simulink library "PCMULib"  (R2022b)
settings: Solver=ode45  StartTime=0.0  StopTime=10.0  RelTol=1e-3  EnableMultiTasking=on
undefined symbols (not defined in the file or in its folder): BreakpointData, BreakpointData1, BreakpointData2, BreakpointData_One_A, BreakpointData_Two_A, caaaa_dbi, caaaa_swi, cTmComprCtrl_n_i16SM4CmpHeatKiMax, cTmComprCtrl_n_i16SM4CmpHeatKiMin, cTmComprCtrl_n_i16SM4CmpHeatKpMax, cTmComprCtrl_n_i16SM4CmpHeatKpMin, cTmComprCtrl_Te_s32ErrCmpPIContinueHeatH, cTmComprCtrl_Te_s32ErrCmpPIContinueHeatL, cTmIn_n_ElacCmprReq_db, cTmIn_n_ElacCmprReq_sw, db, dbi, E2E_P01DataIDMode, E2E_P01ReceiverStatusType, EnumClass, iBit, initalValue, No_Runnable_Period, ObB_EidBsgStDerat_C, p_OVERRIDE_MASTER_SWITCH, SlDemoSign, sw, swi, SwitchOff_P, SwitchOn_P, Table, TableData_M, VCCTi33, VSysD_FidVehDerat1_C
libraries: simulink x22, CCMLib x11, simulink_need_slupdate x9, UXFD_Lib x7, canmsglib x2, PTCC_Lib x1, hdlsllib x1
(part 4 of 7)

== system PCMULib/Standard/Calibration ==
  note: Look-up masks including
      | lookup and prelookup blocks
  note: Look-up and pre-lookup blocks
  note: Calibration
  note: OverRide
  1-D Lookup Table : Lookup  InputValues=BreakpointData  Table=Table  LookUpMeth=Interpolation-Use End Values  OutDataTypeStr=single  SaturateOnIntegerOverflow=off
      settings: CopyFcn=set_param(gcbh,'ShowName','on');
  1-D Lookup Table Without Const_Param : Subsystem  Tag=AVLib calibration  mask(Lookup Table 1D){BlockConfiguration=freeze, BreakpointData=BreakpointData, ReferenceBreakpointData=off, OpenMPTBreakpointData=off, OpenADDBreakpointData=off, IndexSearchMethod=Linear search, Table=Table, ReferenceTable=off, OpenMPTTable=off, OpenADDTable=off, InterpMethod=Linear, DisplayCalibrationNames=off, AdoptBlockName=off, OutMin=[], OutMax=[], OutDataType=Inherit: Inherit from data, IndexDataType=uint8, FractionDataType=Inherit: Inherit via internal rule}
      mask prompts: BlockConfiguration "Block configuration:"; BreakpointData "Breakpoint data:"; ReferenceBreakpointData "Treat as calibration reference"; OpenMPTBreakpointData "Open breakpoint data"; OpenADDBreakpointData "Open ADD breakpoint data"; IndexSearchMethod "Index search method:"; Table "Table data:"; ReferenceTable "Treat as calibration reference"; OpenMPTTable "Open table data"; OpenADDTable "Open ADD table data"; InterpMethod "Interpolation method:"; DisplayCalibrationNames "Block annotation with calibration data"; AdoptBlockName "Adopt block name from table name"; OutMin "Output minimum:"; OutMax "Output maximum:"; OutDataType "Output data type:"; IndexDataType "Index data type:"; FractionDataType "Fraction data type:"
      mask help: Perform 1-D linear interpolation of input values using the specified table.
      mask init:
      | % get and transmit data type from value
      | if strcmp(OutDataType,'Inherit: Inherit from data')
      |   val = Table;  nam = get_param(gcb,'Table');
      |   if evalin('base',['exist(''',nam,''',''var'')']),  s = evalin('base',nam);
      |     if isa(s,'mpt.Parameter') || isa(s,'Simulink.Parameter') || isa(s,'AVLmpt.Parameter')
      |       valDataType = s.DataType;
      |       if strcmp(valDataType,'auto'), valDataType = 'double'; end
      |     else
      |       valDataType = class(s);
      |     end
      |   else
      |       valDataType = class(val);
      |   end
      |   if strcmp(valDataType,'logical'), valDataType = 'boolean'; end
      |   set_param([gcb,'/Curve'],'OutDataTypeStr',valDataType)
      | end
      | if 1
      |   val = BreakpointData;  nam = get_param(gcb,'BreakpointData');
      |   if evalin('base',['exist(''',nam,''',''var'')']),  s = evalin('base',nam);
      |     if isa(s,'mpt.Parameter') || isa(s,'Simulink.Parameter') || isa(s,'AVLmpt.Parameter')
      |       valDataType = s.DataType;
      |       if strcmp(valDataType,'auto'), valDataType = 'double'; end
      |     else
      |       valDataType = class(s);
      |     end
      |   else
      |       valDataType = class(val);
      |   end
      |   if strcmp(valDataType,'logical'), valDataType = 'boolean'; end
      |   set_param([gcb,'/u'],'OutDataTypeStr',valDataType)
      | end
      | 
      | % © AVL S&F, C.A. Roduner, Nov/18/2009
      | if BlockConfiguration==1 && (~strcmp(get_param(gcb,'LinkStatus'),'resolved') ...
      |   || (~strncmp(get_param(gcb,'Referenceblock'),'AVLib',5) && ~exist('AVLib_Init','file') ) ), return, end
      | AVLib_Init( 'LookupTable1D_init', gcb, ...
      |   BlockConfiguration,IndexSearchMethod,InterpMethod, ...
      |   DisplayCalibrationNames,AdoptBlockName,  ...
      |   BreakpointData,ReferenceBreakpointData,OpenMPTBreakpointData, OpenADDBreakpointData, ...
      |   Table,ReferenceTable,OpenMPTTable,OpenADDTable, ...
      |   IndexDataType, FractionDataType, ...
      |   OutMin,OutMax,OutDataType ...
      | );
      mask Help: eval('try openDocu(gcb), catch try run([fileparts(which(''AVLib'')),''\..\AVLibDocu\openDocu'']), catch errordlg(''No documentation available on Matlab path.'',gcb,''modal''), end, end')
      mask TypeOptions BlockConfiguration: freeze | enable | default
      mask Callback BreakpointData:
      | if strcmp(get_param(gcb,'BlockConfiguration'),'freeze'), return, end
      | AVLib_Init('Calibration_cb',gcb,'BreakpointData')
      mask Callback OpenMPTBreakpointData:
      | if strcmp(get_param(gcb,'BlockConfiguration'),'freeze'), return, end
      | AVLib_Init('OpenMPT_cb',gcb,'BreakpointData')
      mask Callback OpenADDBreakpointData:
      | if strcmp(get_param(gcb,'BlockConfiguration'),'freeze'), return, end
      | if strcmp(get_param(gcb,'OpenADDBreakpointData'),'on')
      |   set_param(gcb,'OpenADDBreakpointData','off')
      |   set_param(gcb,'BreakpointData', connectADD(get_param(gcb,'BreakpointData'),'axis') )
      | end
      mask TypeOptions IndexSearchMethod: Evenly spaced points | Linear search | Binary search
      mask Callback Table:
      | if strcmp(get_param(gcb,'BlockConfiguration'),'freeze'), return, end
      | AVLib_Init('Calibration_cb',gcb,'Table')
      mask Callback OpenMPTTable:
      | if strcmp(get_param(gcb,'BlockConfiguration'),'freeze'), return, end
      | AVLib_Init('OpenMPT_cb',gcb,'Table')
      mask Callback OpenADDTable:
      | if strcmp(get_param(gcb,'BlockConfiguration'),'freeze'), return, end
      | if strcmp(get_param(gcb,'OpenADDTable'),'on')
      |   set_param(gcb,'OpenADDTable','off')
      |   set_param(gcb,'Table', connectADD(get_param(gcb,'Table'),'curve') )
      | end
      mask TypeOptions InterpMethod: None - Flat | Linear
      mask Callback AdoptBlockName:
      | if strcmp(get_param(gcb,'BlockConfiguration'),'freeze'), return, end
      | AVLib_Init('AdoptBlockName_cb',gcb,get_param(gcb,'Table'))
      mask TypeOptions OutDataType: Inherit: Inherit from data | Inherit: Inherit via back propagation | double | single | int8 | uint8 | int16 | uint16 | int32 | uint32 | boolean
      mask TypeOptions IndexDataType: uint8 | uint16 | uint32
      mask TypeOptions FractionDataType: Inherit: Inherit via internal rule | double | single
      mask DialogControl ParameterTabVar0 Prompt: Main
      mask DialogControl ParameterTabVar01 Prompt: Signal Attributes
      mask DialogControl ParameterTabVar012 Prompt: Lookup Attributes
      mask Display:
      | plot( getfield(get_param(gcb,'UserData'),'xy') )
      | plot( getfield(get_param(gcb,'UserData'),'xy_InterpMethod') )
      | color('blue'), plot( getfield(get_param(gcb,'UserData'),'xy_C') )
  2-D Lookup Table : Lookup2D  RowIndex=BreakpointData1  ColumnIndex=BreakpointData2  Table=Table  LookUpMeth=Interpolation-Use End Values  OutDataTypeStr=single  SaturateOnIntegerOverflow=off  InputSameDT=off
      settings: CopyFcn=set_param(gcbh,'ShowName','on');
  2-D Lookup Table Without Const_Param : Subsystem  Tag=AVLib calibration  mask(Lookup Table 2D){BlockConfiguration=freeze, BreakpointData1=BreakpointData1, ReferenceBreakpointData1=off, OpenMPTBreakpointData1=off, OpenADDBreakpointData1=off, BreakpointData2=BreakpointData2, ReferenceBreakpointData2=off, OpenMPTBreakpointData2=off, OpenADDBreakpointData2=off, IndexSearchMethod=Binary search, Table=Table, ReferenceTable=off, OpenMPTTable=off, OpenADDTable=off, InterpMethod=Linear, DisplayCalibrationNames=off, AdoptBlockName=off, OutMin=[], OutMax=[], OutDataType=Inherit: Inherit from data, IndexDataType=uint8, FractionDataType=Inherit: Inherit via internal rule}
      mask prompts: BlockConfiguration "Block configuration:"; BreakpointData1 "Breakpoint data for 1st input (x-axis, row index):"; ReferenceBreakpointData1 "Treat as calibration reference"; OpenMPTBreakpointData1 "Open breakpoint data 1"; OpenADDBreakpointData1 "Open ADD breakpoint data 1"; BreakpointData2 "Breakpoint data for 2nd input (y-axis, column index):"; ReferenceBreakpointData2 "Treat as calibration reference"; OpenMPTBreakpointData2 "Open breakpoint data 2"; OpenADDBreakpointData2 "Open ADD breakpoint data 2"; IndexSearchMethod "Index search method:"; Table "Table data:"; ReferenceTable "Treat as calibration reference"; OpenMPTTable "Open table data"; OpenADDTable "Open ADD table data"; InterpMethod "Interpolation method:"; DisplayCalibrationNames "Block annotation with calibration data"; AdoptBlockName "Adopt block name from table name"; OutMin "Output minimum:"; OutMax "Output maximum:"; OutDataType "Output data type:"; IndexDataType "Index data type:"; FractionDataType "Fraction data type:"
      mask help:
      | Perform 2-D linear interpolation of input values using the specified table.
      | The first dimension corresponds to the top (or left) input.
      mask init:
      | % get and transmit data type from value
      | if strcmp(OutDataType,'Inherit: Inherit from data')
      |   val = Table;  nam = get_param(gcb,'Table');
      |   if evalin('base',['exist(''',nam,''',''var'')']),  s = evalin('base',nam);
      |     if isa(s,'mpt.Parameter') || isa(s,'Simulink.Parameter') || isa(s,'AVLmpt.Parameter')
      |       valDataType = s.DataType;
      |       if strcmp(valDataType,'auto'), valDataType = 'double'; end
      |     else
      |       valDataType = class(s);
      |     end
      |   else
      |       valDataType = class(val);
      |   end
      |   if strcmp(valDataType,'logical'), valDataType = 'boolean'; end
      |   set_param([gcb,'/Map'],'OutDataTypeStr',valDataType)
      | end
      | if 1
      |   val = BreakpointData1;  nam = get_param(gcb,'BreakpointData1');
      |   if evalin('base',['exist(''',nam,''',''var'')']),  s = evalin('base',nam);
      |     if isa(s,'mpt.Parameter') || isa(s,'Simulink.Parameter') || isa(s,'AVLmpt.Parameter')
      |       valDataType = s.DataType;
      |       if strcmp(valDataType,'auto'), valDataType = 'double'; end
      |     else
      |       valDataType = class(s);
      |     end
      |   else
      |       valDataType = class(val);
      |   end
      |   if strcmp(valDataType,'logical'), valDataType = 'boolean'; end
      |   set_param([gcb,'/u1'],'OutDataTypeStr',valDataType)
      | end
      | if 1
      |   val = BreakpointData2;  nam = get_param(gcb,'BreakpointData2');
      |   if evalin('base',['exist(''',nam,''',''var'')']),  s = evalin('base',nam);
      |     if isa(s,'mpt.Parameter') || isa(s,'Simulink.Parameter') || isa(s,'AVLmpt.Parameter')
      |       valDataType = s.DataType;
      |       if strcmp(valDataType,'auto'), valDataType = 'double'; end
      |     else
      |       valDataType = class(s);
      |     end
      |   else
      |       valDataType = class(val);
      |   end
      |   if strcmp(valDataType,'logical'), valDataType = 'boolean'; end
      |   set_param([gcb,'/u2'],'OutDataTypeStr',valDataType)
      | end
      | 
      | % © AVL S&F, C.A. Roduner, Nov/18/2009
      | if BlockConfiguration==1 && (~strcmp(get_param(gcb,'LinkStatus'),'resolved') ...
      |   || (~strncmp(get_param(gcb,'Referenceblock'),'AVLib',5) && ~exist('AVLib_Init','file') ) ), return, end
      | AVLib_Init( 'LookupTable2D_init', gcb, ...
      |   BlockConfiguration,IndexSearchMethod,InterpMethod, ...
      |   DisplayCalibrationNames,AdoptBlockName,  ...
      |   BreakpointData1,ReferenceBreakpointData1,OpenMPTBreakpointData1, OpenADDBreakpointData1, ...
      |   BreakpointData2,ReferenceBreakpointData2,OpenMPTBreakpointData2, OpenADDBreakpointData2, ...
      |   Table,ReferenceTable,OpenMPTTable,OpenADDTable, ...
      |   IndexDataType, FractionDataType, ...
      |   OutMin,OutMax,OutDataType ...
      | );
      mask Help: eval('try openDocu(gcb), catch try run([fileparts(which(''AVLib'')),''\..\AVLibDocu\openDocu'']), catch errordlg(''No documentation available on Matlab path.'',gcb,''modal''), end, end')
      mask TypeOptions BlockConfiguration: freeze | enable | default
      mask Callback BreakpointData1:
      | if strcmp(get_param(gcb,'BlockConfiguration'),'freeze'), return, end
      | AVLib_Init('Calibration_cb',gcb,'BreakpointData1')
      mask Callback OpenMPTBreakpointData1:
      | if strcmp(get_param(gcb,'BlockConfiguration'),'freeze'), return, end
      | AVLib_Init('OpenMPT_cb',gcb,'BreakpointData1')
      mask Callback OpenADDBreakpointData1:
      | if strcmp(get_param(gcb,'BlockConfiguration'),'freeze'), return, end
      | if strcmp(get_param(gcb,'OpenADDBreakpointData1'),'on')
      |   set_param(gcb,'OpenADDBreakpointData1','off')
      |   set_param(gcb,'BreakpointData1', connectADD(get_param(gcb,'BreakpointData1'),'axis1') )
      | end
      mask Callback BreakpointData2:
      | if strcmp(get_param(gcb,'BlockConfiguration'),'freeze'), return, end
      | AVLib_Init('Calibration_cb',gcb,'BreakpointData2')
      mask Callback OpenMPTBreakpointData2:
      | if strcmp(get_param(gcb,'BlockConfiguration'),'freeze'), return, end
      | AVLib_Init('OpenMPT_cb',gcb,'BreakpointData2')
      mask Callback OpenADDBreakpointData2:
      | if strcmp(get_param(gcb,'BlockConfiguration'),'freeze'), return, end
      | if strcmp(get_param(gcb,'OpenADDBreakpointData2'),'on')
      |   set_param(gcb,'OpenADDBreakpointData2','off')
      |   set_param(gcb,'BreakpointData2', connectADD(get_param(gcb,'BreakpointData2'),'axis2') )
      | end
      mask TypeOptions IndexSearchMethod: Evenly spaced points | Linear search | Binary search
      mask Callback Table:
      | if strcmp(get_param(gcb,'BlockConfiguration'),'freeze'), return, end
      | AVLib_Init('Calibration_cb',gcb,'Table')
      mask Callback OpenMPTTable:
      | if strcmp(get_param(gcb,'BlockConfiguration'),'freeze'), return, end
      | AVLib_Init('OpenMPT_cb',gcb,'Table')
      mask Callback OpenADDTable:
      | if strcmp(get_param(gcb,'BlockConfiguration'),'freeze'), return, end
      | if strcmp(get_param(gcb,'OpenADDTable'),'on')
      |   set_param(gcb,'OpenADDTable','off')
      |   set_param(gcb,'Table', connectADD(get_param(gcb,'Table'),'map') )
      | end
      mask TypeOptions InterpMethod: None - Flat | Linear
      mask Callback AdoptBlockName:
      | if strcmp(get_param(gcb,'BlockConfiguration'),'freeze'), return, end
      | AVLib_Init('AdoptBlockName_cb',gcb,get_param(gcb,'Table'))
      mask TypeOptions OutDataType: Inherit: Inherit from data | Inherit: Inherit via back propagation | double | single | int8 | uint8 | int16 | uint16 | int32 | uint32 | boolean
      mask TypeOptions IndexDataType: uint8 | uint16 | uint32
      mask TypeOptions FractionDataType: Inherit: Inherit via internal rule | double | single
      mask DialogControl ParameterTabVar0 Prompt: Main
      mask DialogControl ParameterTabVar01 Prompt: Signal Attributes
      mask DialogControl ParameterTabVar012 Prompt: Lookup Attributes
      mask Display:
      | port_label('input',1,'x'), port_label('input',2,'y')
      | plot( getfield(get_param(gcb,'UserData'),'xy') )
      | plot( getfield(get_param(gcb,'UserData'),'xy_InterpMethod') )
      | color('blue'), plot( getfield(get_param(gcb,'UserData'),'xy_C') )
  Interpolation Using Prelookup : Interpolation_n-D  InternalRulePriority=Speed
      settings: CopyFcn=set_param(gcbh,'ShowName','off');
  OverRide : Subsystem  mask(override){}
      settings: CopyFcn=set_param(gcbh,'ShowName','off');
  OverRide_with_master_switch : Subsystem  mask(override){}
      settings: CopyFcn=set_param(gcbh,'ShowName','off');
  Parameter : Constant  Value=Parameter
      settings: CopyFcn=set_param(gcbh,'ShowName','off');
  Prelookup : PreLookup  BreakpointsData=[10:10:110]  ExtrapMethod=Linear
      settings: CopyFcn=set_param(gcbh,'ShowName','off');
  SwitchState : Relay  OnSwitchValue=SwitchOn_P  OffSwitchValue=SwitchOff_P
      settings: CopyFcn=set_param(gcbh,'ShowName','on');
      settings: AttributesFormatString=|
      | %<OnSwitchValue>
      | %<OffSwitchValue>
  n-D Lookup Table : Lookup_n-D  BreakpointsForDimension1=BreakpointData_One_A  BreakpointsForDimension2=BreakpointData_Two_A  Table=TableData_M  ExtrapMethod=Clip  UseLastTableValue=on  InternalRulePriority=Speed  RndMeth=Simplest  SaturateOnIntegerOverflow=on
      settings: CopyFcn=set_param(gcbh,'ShowName','on');  InputPortMap=u0,u1
  xbackground1 : Subsystem
      settings: CopyFcn=set_param(gcbh,'ShowName','off');
      mask Display: disp(' ')
  xbackground2 : Subsystem
      settings: CopyFcn=set_param(gcbh,'ShowName','off');
      mask Display: disp(' ')
  xbackground3 : Subsystem
      settings: CopyFcn=set_param(gcbh,'ShowName','off');
      mask Display: disp(' ')
  xbackground4 : Subsystem
      settings: CopyFcn=set_param(gcbh,'ShowName','off');
      mask Display: disp(' ')

== system PCMULib/Standard/Discrete dynamics ==
  note: Hystresis filter
  note: Bumpless transfer
  note: Unit delay
  note: Discrete
      | derivate
  note: Rate limiter
  note: First order filters (VCC)
  note: Second order filters(VCC)
  BumplessRateTransfer : Subsystem  mask(VCC_BumplessTransferRate_1.0){}
      mask help:
      | Makes a bumpless rate transfer from u2  to u1
      | when s goes from 0 to 1. It is very important that
      |  the Trig signal assumes the values <= 0 and >= 1.
      | The transfer happens during a time controlled by a
      | filter with a time constant that can be calibrated.
      settings: CopyFcn=set_param(gcbh,'ShowName','off');
      mask Display:
      | plot([0.2 1], [0.2 0.2]);
      | plot([0.2 0.3], [0.22 0.22]);
      | plot([0.7 1], [0.78 0.78]);
      | plot([0.2 1], [0.8 0.8]);
      | plot([0.7 1], [0.78 0.78]);
      | plot([0.3 0.7],[0.22, 0.78])
      | plot([0.38, 0.5, 0.52], [0.46, 0.5, 0.37])
  BumplessTransfer : Subsystem  mask(GL_BumplessTransferFilter_1.0){}
      mask help:
      | Makes a bumpless transfer from u2  to u1
      | when s goes from 0 to 1. It is very important that
      |  the Trig signal assumes the values <= 0 and >= 1.
      | The transfer happens during a time controlled by a
      | filter with a time constant that can be calibrated.
      mask init:
      | set_param(gcb,'LinkStatus','none');
      settings: CopyFcn=set_param(gcbh,'ShowName','off');
      mask Display:
      | plot([0.15 1], [0.2 0.2]);
      | plot([0.15 1], [0.8 0.8]);
      | plot([0.00 0.50 1.00 1.50 2.00 2.50 3.00 ]/3*0.7+0.3, ...
      |      [0.20 0.52 0.67 0.74 0.77 0.79 0.79]);
      | 
      | plot([0.28, 0.4, 0.47], [0.48, 0.5, 0.42])
  DLPF1_pole_v2 : Subsystem  mask(GL_DiscreteDerivative_1.0){}
      mask help:
      | Discrete derivative and low-pass filter. Corresponding analogue transfer function:
      |   s / (1 + tc * s)
      mask init:
      | set_param(gcb,'LinkStatus','none');
      settings: CopyFcn=set_param(gcbh,'ShowName','off');
      mask Display:
      | plot([0.35, 0.9], [0, 0], [0.35, 0.35], [0, 1])
      | plot(0.35:0.55/10:0.9,  1- [0 0.39 0.63 0.78 0.86 0.92 0.95 0.97 0.98 0.99 0.99])
  FirstOrderFilter : Subsystem  mask(VCC_FirstOrderFilter_1.0){}
      mask help: Discrete low-pass filter. Corresponding analogue transfer function: 1 / (1 + tc * s)
      settings: CopyFcn=set_param(gcbh,'ShowName','on');
      mask Display:
      | plot([0.35, 0.9], [0, 0], [0.35, 0.35], [0, 1])
      | plot(0.35:0.55/10:0.9,   [0 0.39 0.63 0.78 0.86 0.92 0.95 0.98 0.99 0.99 0.99])
  FirstOrderFilter1 : Subsystem  mask(VCC_FirstOrderFilterExtraFeat_1.0){}
      mask help:
      | Discrete low-pass filter. Corresponding analogue transfer function: 1 / (1 + tc * s)
      |
      | Parameters:
      | Error - An output which shows the difference between the input and output signal values
      | Different increase and decrease tc -
      | Reset - Sets the output value = rv when r = 1
      settings: CopyFcn=set_param(gcbh,'ShowName','on');
      mask Display:
      | plot([0.35, 0.9], [0, 0], [0.35, 0.35], [0, 1])
      | plot(0.35:0.55/10:0.9,   [0 0.39 0.63 0.78 0.86 0.92 0.95 0.98 0.99 0.99 0.99])
  HysteresisFilter : Subsystem  mask(GL_HysteresisFilter_1.0){}
      mask help:
      | Filter to avoid occilation during low slipp
      | when converter character is steep
      mask init:
      | set_param(gcb,'LinkStatus','none');
      settings: CopyFcn=set_param(gcbh,'ShowName','off');
      mask Display:
      | text(0.1, 0.8, 'u');
      | text(0.1, 0.3, 'h');
      | plot([0.3, 0.6, 0.9], [0.1, 0.1, 0.9]);
      | plot([0.3, 0.6, 0.9], [0.1, 0.9, 0.9]);
      | plot([0.4, 0.55], [0.4, 0.4]);
      | plot([0.7, 0.84], [0.7, 0.7]);
  LPF1_discreteReset : Subsystem  Description=|  mask(PAG_FirstOrder_Smoothing_Filter_Reset_LV1.8_BV5){OpenTL=Select block:, OutputLineName=}
      | Purpose Use the block to implement a discrete low pass filter.
      | 
      | When the input signal r is TRUE the output will assume the
      | value of the input signal. This is used to set initial values of
      | the filter.
      | 
      | Difference to Simulink and justification
      | Additional block to perform special feature for ECM implementation
      | in a standard manner. Block name hidden, since icon clearly conveys
      | meaning and name adds unnecessary clutter to the page.
      mask prompts: OpenTL "Open Target Link dialog"; OutputLineName "Output line name"
      mask help:
      | Discrete first order low pass filter. Discrete transfer function:
      | y(k)=a*y(k-1)+(1-a)*u(k)
      | When the input signal r is TRUE the output will assume the
      | value of the input signal. This is used to set initial values of
      | the filter.
      mask init:
      | %% Reset the opendialog popupvalue
      | Values=get_param(gcbh,'maskvalues');
      | Values{1}='Select block:';
      | set_param(gcbh,'maskvalues',Values);
      | 
      | %Set the line name, 
      | CurrentBlock=gcbh;
      | %Find the output variable block
      | while strcmp(get_param(CurrentBlock,'blocktype'),'SubSystem')
      |     Tmp=get_param(find_system(CurrentBlock,'lookundermasks','on','searchdepth',1,'blocktype','Outport','Port','1'),'linehandles');
      |     CurrentBlock=get_param(Tmp.Inport,'srcblockhandle');
      | end
      | set_param(Tmp.Inport,'name',get_param(gcbh,'OutputLineName'));
      | 
      | 
      | %% Adjust the propagated output line name
      | Tmp=get_param(gcbh,'linehandles');
      | OutputLine=Tmp.Outport;
      | if OutputLine~=-1
      |     
      |     if isempty(get_param(gcbh,'OutputLineName'))
      |         set(OutputLine,'signalPropagation','off')
      |         set(OutputLine,'name','')
      |     else
      |         set(OutputLine,'name',['<' get_param(gcbh,'OutputLineName') '>'])
      |     end
      | end
      settings: CopyFcn=set_param(gcbh,'ShowName','on');
      mask TypeOptions OpenTL: Select block: | Output variable
      mask Callback OpenTL:
      | if strcmp(get_param(gcbh,'OpenTL'),'Output variable')
      |     BlockType='SubSystem';
      |     OutputVariableBlock=gcbh;
      |     while strcmp(BlockType,'SubSystem');
      |     Tmp=get_param(find_system(OutputVariableBlock,'lookundermasks','on','searchdepth',1,'blocktype','Outport','Port','1'),'linehandles');
      |     OutputVariableBlock=get_param(Tmp.Inport,'srcblockhandle');
      |     BlockType=get_param(OutputVariableBlock,'blocktype');
      |     end
      | 
      |     MaskType=get_param(OutputVariableBlock,'masktype');
      |     if strmatch('TL',MaskType)
      | 
      |         if ismember(MaskType,{'TL_Sum','TL_Product'})
      |             MaskName='tl_sumprod_dlg';
      |         elseif ismember(MaskType,{'TL_LogicalOperator','TL_RelationalOperator'})
      |             MaskName='tl_rel_dlg';
      |         elseif strcmp(MaskType,'TL_MinMax')
      |             MaskName='tl_minmax_dlg';
      |         elseif strcmp(MaskType,'TL_Gain')
      |             MaskName='tl_gain_dlg';
      |         elseif strcmp(MaskType,'TL_Switch')
      |             MaskName='tl_switch_dlg';
      |         end
      | 
      |         dstabdlg('create',MaskName,OutputVariableBlock);
      |     end
      | end
      mask Display:
      | plot([0.3, 1], [0, 0], [0.3, 0.3], [0, 1])
      | plot([0 0.1 0.1 0.2 0.2 0.3 0.3 0.4 0.4 0.5 0.5 0.6 0.6 0.7 0.7 0.8 0.8 0.9 0.9 1 1]*0.7+0.3, [ 0 0 0.39 0.39 0.63 0.63 0.78 0.78 0.86 0.86 0.92 0.92 0.95 0.95 0.97 0.97 0.98 0.98 0.99 0.99 0.99])
  LPF2_discrete : Subsystem  mask(PAG_SecondOrder_Discrete_Filter_LV1.8_BV3){OpenTL=Select block:, OutputLineName=}
      mask prompts: OpenTL "Open Target Link dialog"; OutputLineName "Output line name"
      mask help:
      | Discrete  filter.
      |
      | y(k) = -a1 y(k-1) - a2 y(k-2) + b0 u(k) + b1 u(k-1) + b2 u(k-2)
      mask init: same as PCMULib/Standard/Discrete dynamics/LPF1_discreteReset
      settings: CopyFcn=set_param(gcbh,'ShowName','off');
      mask TypeOptions OpenTL: Select block: | Output variable
      mask Callback OpenTL:
      | if strcmp(get_param(gcbh,'OpenTL'),'Output variable')
      |     BlockType='SubSystem';
      |     OutputVariableBlock=gcbh;
      |     while strcmp(BlockType,'SubSystem');
      |     Tmp=get_param(find_system(OutputVariableBlock,'lookundermasks','on','searchdepth',1,'blocktype','Outport','Port','1'),'linehandles');
      |     OutputVariableBlock=get_param(Tmp.Inport,'srcblockhandle');
      |     BlockType=get_param(OutputVariableBlock,'blocktype');
      |     end
      | 
      |     MaskType=get_param(OutputVariableBlock,'masktype');
      |     if strmatch('TL',MaskType)
      | 
      |         if ismember(MaskType,{'TL_Sum','TL_Product'})
      |             MaskName='tl_sumprod_dlg';
      |         elseif ismember(MaskType,{'TL_LogicalOperator','TL_RelationalOperator'})
      |             MaskName='tl_rel_dlg';
      |         elseif strcmp(MaskType,'TL_MinMax')
      |             MaskName='tl_minmax_dlg';
      |         elseif strcmp(MaskType,'TL_Gain')
      |             MaskName='tl_gain_dlg';
      |         elseif strcmp(MaskType,'TL_Switch')
      |             MaskName='tl_switch_dlg';
      |         end
      | 
      |         dstabdlg('create',MaskName,OutputVariableBlock);
      |     end
      | end
      mask Display:
      | plot([0.45, 1], [0, 0], [0.45, 0.45], [0, 1])
      | plot([0 0.1 0.1 0.2 0.2 0.3 0.3 0.4 0.4 0.5 0.5 0.6 0.6 0.7 0.7 0.8 0.8 0.9 0.9 1 1]*0.55+0.45, [ 0 0 0.39 0.39 0.63 0.63 0.78 0.78 0.86 0.86 0.92 0.92 0.95 0.95 0.97 0.97 0.98 0.98 0.99 0.99 0.99])
  LPF2_omega : Subsystem  mask(PAG_SecondOrder_Filter_LV1.8_BV4){OpenTL=Select block:, OutputLineName=}
      mask prompts: OpenTL "Open Target Link dialog"; OutputLineName "Output line name"
      mask help:
      | An Euler discretization of a filter with transfer function
      |                          2
      |                       w
      | G(s) = -----------------------------
      |              2                     2
      |            s  + 2 w z s + w
      mask init: same as PCMULib/Standard/Discrete dynamics/LPF1_discreteReset
      settings: CopyFcn=set_param(gcbh,'ShowName','off');
      mask TypeOptions OpenTL: Select block: | Output variable
      mask Callback OpenTL:
      | if strcmp(get_param(gcbh,'OpenTL'),'Output variable')
      |     BlockType='SubSystem';
      |     OutputVariableBlock=gcbh;
      |     while strcmp(BlockType,'SubSystem');
      |     Tmp=get_param(find_system(OutputVariableBlock,'lookundermasks','on','searchdepth',1,'blocktype','Outport','Port','1'),'linehandles');
      |     OutputVariableBlock=get_param(Tmp.Inport,'srcblockhandle');
      |     BlockType=get_param(OutputVariableBlock,'blocktype');
      |     end
      | 
      |     MaskType=get_param(OutputVariableBlock,'masktype');
      |     if strmatch('TL',MaskType)
      | 
      |         if ismember(MaskType,{'TL_Sum','TL_Product'})
      |             MaskName='tl_sumprod_dlg';
      |         elseif ismember(MaskType,{'TL_LogicalOperator','TL_RelationalOperator'})
      |             MaskName='tl_rel_dlg';
      |         elseif strcmp(MaskType,'TL_MinMax')
      |             MaskName='tl_minmax_dlg';
      |         elseif strcmp(MaskType,'TL_Gain')
      |             MaskName='tl_gain_dlg';
      |         elseif strcmp(MaskType,'TL_Switch')
      |             MaskName='tl_switch_dlg';
      |         end
      | 
      |         dstabdlg('create',MaskName,OutputVariableBlock);
      |     end
      | end
      mask Display:
      | plot([0.45, 0.9], [0, 0], [0.45, 0.45], [0, 1])
      | plot(0.45:0.45/10:0.9,   [ 0 0.05 0.1 0.8 1.0 0.95 0.85 0.9 0.95 0.92 0.9 ])
  RateLimit : Subsystem  mask(GL_RateLimiter_1.0){}
      mask help: Rate limiter. Limits the derivative of the input signal to the input value d.
      mask init:
      | set_param(gcb,'LinkStatus','none');
      settings: CopyFcn=set_param(gcbh,'ShowName','off');
      mask Display:
      | plot([0.35, 0.55, 0.55, 1.0], [0, 0, 1, 1])
      | plot([0.35, 0.55, 0.8, 1.0], [0, 0, 1, 1])
  RateLimit1 : Subsystem  mask(GL_RateLimiterExtraFeat_1.0){}
      mask help:
      | Rate limiter. Limits the derivative of the input signal to the input value d.
      |
      | Parameters:
      | Different increase and decrease rate -
      | Reset - Sets the output value = rv when r = 1
      mask init:
      | set_param(gcb,'LinkStatus','none');
      settings: CopyFcn=set_param(gcbh,'ShowName','off');
      mask Display:
      | plot([0.35, 0.55, 0.55, 1.0], [0, 0, 1, 1])
      | plot([0.35, 0.55, 0.8, 1.0], [0, 0, 1, 1])
  Unit Delay : UnitDelay  SampleTime=-1  HasFrameUpgradeWarning=on
      settings: CopyFcn=set_param(gcbh,'ShowName','off');
  xbackground1 : Subsystem
      settings: CopyFcn=set_param(gcbh,'ShowName','off');
      mask Display: disp(' ')
  xbackground2 : Subsystem
      settings: CopyFcn=set_param(gcbh,'ShowName','off');
      mask Display: disp(' ')
  xbackground3 : Subsystem
      settings: CopyFcn=set_param(gcbh,'ShowName','off');
      mask Display: disp(' ')
  xbackground4 : Subsystem
      settings: CopyFcn=set_param(gcbh,'ShowName','off');
      mask Display: disp(' ')
  xbackground5 : Subsystem
      settings: CopyFcn=set_param(gcbh,'ShowName','off');
      mask Display: disp(' ')
  xbackground6 : Subsystem
      settings: CopyFcn=set_param(gcbh,'ShowName','off');
      mask Display: disp(' ')
  xbackground7 : Subsystem
      settings: CopyFcn=set_param(gcbh,'ShowName','off');
      mask Display: disp(' ')

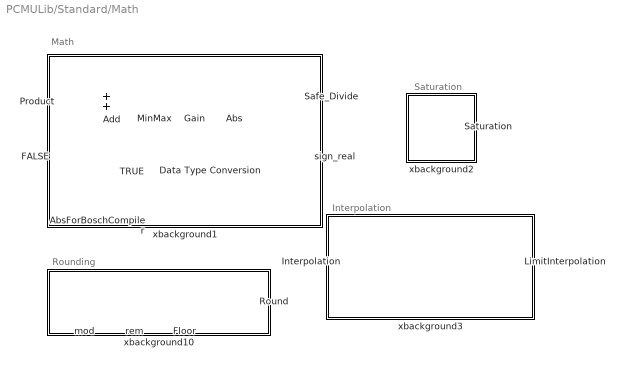
== system PCMULib/Standard/Math ==
  note: Interpolation
  note: Rounding
  note: Math
  note: Saturation
  Abs : Abs  SaturateOnIntegerOverflow=off
      settings: CopyFcn=set_param(gcbh,'ShowName','off');
  AbsForBoschCompiler : Subsystem  mask(VCC_Abs_1.0){}
      mask help: y=|u|
      mask Display: disp('|u|')
  Add : Sum
      settings: CopyFcn=set_param(gcbh,'ShowName','off');
  Data Type Conversion : DataTypeConversion  SaturateOnIntegerOverflow=off  RndMeth=Floor
      settings: CopyFcn=set_param(gcbh,'ShowName','off');
  FALSE : Constant  ClipboardFcn="href=\"http://183.136.146.131:8080/redmine/my/page\";"  Value=false
      settings: CopyFcn=set_param(gcbh,'ShowName','off');  OpenFcn="href=\"http://183.136.146.131:8080/redmine/my/page\";"
  Floor : Subsystem  mask(GL_Floor){}
      mask help: Floor block rounds the input variable to the nearest integer towards minus infinity.
      settings: CopyFcn=set_param(gcbh,'ShowName','off');
      mask Display: text(0.1,0.5, 'Floor')
  Gain : Gain
      settings: CopyFcn=set_param(gcbh,'ShowName','off');
  Interpolation : Subsystem  mask(GL_Interpolation_1.0){}
      mask help: Linear interpolation. The output is given by y=k(u-x1)+y1, where k=(y2-y1)/(x2-x1)
      settings: CopyFcn=set_param(gcbh,'ShowName','on');
      mask Display:
      | plot([0.2, 0.9], [0.2, 0.2]);
      | plot([0.2, 0.2], [0.2, 0.9]);
      | plot([0.4,  0.6], [0.25, 0.85]);
      | text(0.40, 0.27, '(x1, y1)');
      | text(0.50, 0.88, '(x2, y2)');
  LimitInterpolation : Subsystem  mask(GL_LimitInterpolation_1.0){}
      mask help:
      | Interpolation with limitations.  The output is given by  y=k(u-x1)+y1, where k=(y2-y1)/(x2-x1)
      | The output value is also limited to the interval  y1 < y < y2.
      settings: CopyFcn=set_param(gcbh,'ShowName','on');
      mask Display:
      | plot([0.2, 0.9], [0.2, 0.2]);
      | plot([0.2, 0.2], [0.2, 0.9]);
      | plot([0.25, 0.4,  0.6, 0.85], [0.25, 0.25, 0.85, 0.85]);
      | text(0.40, 0.27, '(x1,  y1)');
      | text(0.50, 0.88, '(x2,  y2)');
  MinMax : MinMax
      settings: CopyFcn=set_param(gcbh,'ShowName','off');
  Product : Product
      settings: CopyFcn=set_param(gcbh,'ShowName','off');
  Round : Subsystem  mask(GL_Round){}
      mask help: Rounds to nearest integer
      settings: CopyFcn=set_param(gcbh,'ShowName','off');
      mask Display: text(0.1,0.5, 'Round')
  Safe_Divide : Subsystem  mask(GL_SafeDivide_1.0){}
      mask help:
      | Safe Divide, prevents division by zero.
      |
      | if abs(denominator) > eps then
      |     output = numerator / denominator
      | else
      |     output = numerator / eps
      |
      | Attention!
      | Use this block only when there is a risk for division by zero.
      mask Display:
      | port_label('input', 1, 'x')
      | port_label('input', 2, '÷')
      | port_label('input', 3, 'eps')
  Saturation : Subsystem  mask(GL_Saturation_1.0){}
      mask help:
      | If input_1 > input_2
      |   output = input_2
      | elseif input_1 < input_3
      |   output = input_3
      | else
      |   output = input_1
      |
      | Note that if the lower limit is set above the upper limit, the output will take the value of the input to the lower limit port.
      settings: CopyFcn=set_param(gcbh,'ShowName','off');
      mask Display: plot([0.3, 0.5, 0.7, 0.9], [0, 0, 1, 1])
  TRUE : Constant  Value=true
      settings: CopyFcn=set_param(gcbh,'ShowName','off');
  mod : Subsystem  mask(GL_Mod_1.0){}
      mask help: Signed remainder after division.
      settings: CopyFcn=set_param(gcbh,'ShowName','off');
      mask Display: disp('mod')
  rem : Subsystem  mask(GL_Rem_1.0){}
      mask help: Remainder after division.
      settings: CopyFcn=set_param(gcbh,'ShowName','off');
      mask Display: disp('rem')
  sign_real : Subsystem
      mask Display:
      | text(0.18, 0.275, '-1');
      | text(0.75, 0.75, '1');
      | text(0.55, 0.42, '0');
      | plot([0.25, 0.5, 0.5, 0.75],[0.25, 0.25, 0.75, 0.75])
      | plot([0,1],[0.5, 0.5])
      | plot([0.5,0.5],[0,1])
  xbackground1 : Subsystem
      mask Display: disp(' ')
  xbackground10 : Subsystem
      mask Display: disp(' ')
  xbackground2 : Subsystem
      mask Display: disp(' ')
  xbackground3 : Subsystem
      mask Display: disp(' ')

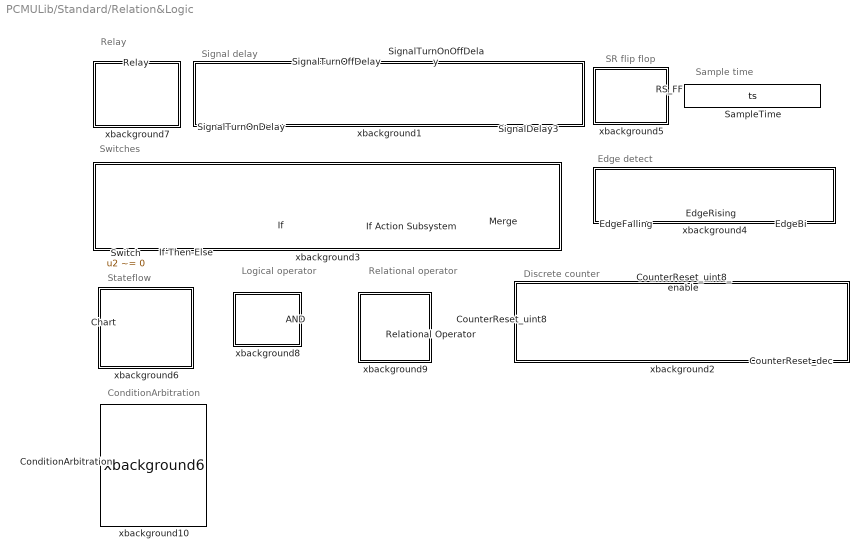
== system PCMULib/Standard/Relation&Logic ==
  note: Relay
  note: Signal delay
  note: Edge detect
  note: Switches
  note: SR flip flop
  note: Stateflow
  note: Logical
      | operator
  note: Relational
      |  operator
  note: Discrete counter
  note: Sample time
  note: ConditionArbitration
  AND : Logic  AllPortsSameDT=off  OutDataTypeStr=boolean
      settings: CopyFcn=set_param(gcbh,'ShowName','off');
  Chart : Stateflow chart  TreatAsAtomicUnit=on
      settings: CopyFcn=set_param(gcbh,'ShowName','off');
  ConditionArbitration : Subsystem  mask(ConditionArbitration){}
      mask help:
      | If Condition1 == Condition2 == 0
      |   Val_0_0 send out
      | elseif Condition1== 0 && Condition2 == 1
      |   Val_0_1 send out
      | elseif Condition1== 1 && Condition2 == 0
      |   Val_1_0 send out
      | else
      |   Val_1_1 send out
      mask Display:
      | port_label('input', 1, 'Condition1');
      | port_label('input', 2, 'Condition2');
      | port_label('input', 3, '0 0');
      | port_label('input', 4, '0 1');
      | port_label('input', 5, '1 0');
      | port_label('input', 6, '1 1');
      | port_label('output', 1, 'out');
  CounterReset_dec : Subsystem  mask(GL_DecreseCounterEnableReset_1.0){}
      mask help:
      | Resetable counter.
      |
      | If r = 1 the counter resets to rv.
      | If r = 0 the block adds/subtracts inc/dec to the output each sample.
      |
      | To count time let inc/dec = sample_time
      | To count samples let inc/dec = 1
      |
      | Enable: Enables the counter if e = 1
      | Dec: Counts down instead of up. Stops counting when output = 0
      settings: CopyFcn=set_param(gcbh,'ShowName','off');
      mask Display:
      | plot([ 0.5 1 1 2 2 3 3 4 4 5 5 6 6 7 7]/14+0.4, ...
      |        [ 0 0 4 4 3 3 2 2 1 1 0 0 0 0 0]/5+0.1)
  CounterReset_uint8 : Subsystem  mask(GL_CounterReset_1.0){}
      mask help:
      | Resetable counter.
      |
      | If r = 1 the counter resets to rv.
      | If r = 0 the block adds/subtracts inc/dec to the output each sample.
      |
      | To count time let inc/dec = sample_time
      | To count samples let inc/dec = 1
      |
      | Enable: Enables the counter if e = 1
      | Dec: Counts down instead of up. Stops counting when output = 0
      settings: CopyFcn=set_param(gcbh,'ShowName','off');
      mask Display: plot([0 1 1 2 2 3 3 4 4 5]/14+0.4, [0 0 1 1 2 2 3 3 4 4]/5+0.1)
  CounterReset_uint8_enable : Subsystem  mask(VCC_CounterEnableReset_1.0){}
      mask help:
      | Resetable counter.
      |
      | If r = 1 the counter resets to rv.
      | If r = 0 the block adds/subtracts inc/dec to the output each sample.
      |
      | To count time let inc/dec = sample_time
      | To count samples let inc/dec = 1
      |
      | Enable: Enables the counter if e = 1
      | Dec: Counts down instead of up. Stops counting when output = 0
      settings: CopyFcn=set_param(gcbh,'ShowName','off');
      mask Display: plot([0 1 1 2 2 3 3 4 4 5]/14+0.4, [0 0 1 1 2 2 3 3 4 4]/5+0.1)
  EdgeBi : Subsystem  mask(GL_EdgeDetectEither_1.0){}
      mask help: Output is 1 of negative or positive edge is detected, otherwise its 0.
      settings: CopyFcn=set_param(gcbh,'ShowName','off');
      mask Display:
      | plot([0 0.5 0.5 1.5 1.5 2], [0 0 1 1 0 0])
      | 
      | patch([0 1 0.5 0], [0.25 0.25 0.85 0.25])
      | patch([1 2 1.5 1], [0.75 0.75 0.15 0.75])
  EdgeFalling : Subsystem  mask(GL_EdgeDetectNegative_1.0){}
      mask help: Output is 1 of negative edge is detected, otherwise its 0.
      settings: CopyFcn=set_param(gcbh,'ShowName','off');
      mask Display:
      | plot([0 0.5 0.5 1.5 1.5 2], [0 0 1 1 0 0])
      | patch([1 2 1.5 1], [0.75 0.75 0.15 0.75])
  EdgeRising : Subsystem  mask(GL_EdgeDetectPositive_1.0){}
      mask help: Output is 1 of positive edge is detected, otherwise its 0.
      settings: CopyFcn=set_param(gcbh,'ShowName','off');
      mask Display:
      | plot([0 0.5 0.5 1.5 1.5 2], [0 0 1 1 0 0])
      | 
      | patch([0 1 0.5 0], [0.25 0.25 0.85 0.25])
  If : If
      settings: CopyFcn=set_param(gcbh,'ShowName','off');
  If Action Subsystem : Subsystem  TreatAsAtomicUnit=on
      settings: CopyFcn=|
      | set_param(gcbh,'ShowName','off');
      | set_param(gcbh,'LinkStatus','none');
  If-Then-Else : Subsystem
      mask Display:
      | port_label('input',1,'If')
      | port_label('input',2,'Then')
      | port_label('input',3,'Else')
  Merge : Merge
      settings: CopyFcn=set_param(gcbh,'ShowName','off');
  RS_FF : Subsystem  mask(GL_SRFlipFlop_1.0){}
      mask help:
      | Set/Reset flip flop.
      |
      |   R   S   Q
      |   1   X   0            (X :  0 or 1)
      |   0   1   1            (P:   keeps previous value)
      |   0   0   P
      settings: CopyFcn=set_param(gcbh,'ShowName','off');
  Relational Operator : RelationalOperator  Operator=<=  OutDataTypeStr=boolean  InputSameDT=off
      settings: CopyFcn=set_param(gcbh,'ShowName','off');
  Relay : Subsystem  mask(GL_Relay_1.0){}
      mask help: Output 1 or 0 ('on' or 'off') by comparing the first input to the thresholds specified by thesecond and third input. The switch on point is specified by the second input and the switch off point is specified by the third input. If the second input becomes less then the third input the relay switch off. The on/off state of the relay is not affected by input between the upper and lower limits.
      settings: CopyFcn=set_param(gcbh,'ShowName','off');
      mask Display: plot( [0.4 0.8 0.8], [0.05  0.05 0.8], [0.6 0.6 0.9], [0.05 0.8 0.8])
  SampleTime : DataStoreMemory  DataStoreName=ts  InitialValue=0.01  ShowAdditionalParam=off  OutDataTypeStr=single  mask(DataStoreMemory){data={'output',{'description',['Sample time'],'name','ts','class','STATIC_MACRO','type','Float32','unit','s'},'date',735300.29223179398}}
      settings: CopyFcn=set_param(gcbh,'ShowName','off');
      mask Display: plot([-0.05, 1.05, NaN, -0.05, 1.05],[.01, .01, NaN, .99, .99])
  SignalDelay3 : Subsystem  mask(GL_SignalDelayEither_1.0){}
      mask help: Signal delay. Delays a logical change the time td. The output signal will not change unless the input signal keeps its value during the time td.
      settings: CopyFcn=set_param(gcbh,'ShowName','off');
      mask Display:
      | plot([0.4 0.7 0.7 0.8], [0.3 0.3 0.7 0.7]+0.3)
      | plot([0.4 0.7 0.7 0.8], [0.7 0.7 0.3 0.3]-0.3)
  SignalTurnOffDelay : Subsystem  mask(VCC_SignalDelayNegative_1.0){}
      mask help: Signal delay. Delays a negative logical change the time td. The output signal will not change unless the input signal keeps its value during the time td.
      mask init:
      | set_param(gcb,'LinkStatus','none');
      settings: CopyFcn=set_param(gcbh,'ShowName','off');
      mask Display: plot([0.4 0.7 0.7 0.8], [0.7 0.7 0.3 0.3])
  SignalTurnOnDelay : Subsystem  mask(GL_SignalDelayPositive_1.0){}
      mask help: Signal delay. Delays a positive logical change the time td. The output signal will not change unless the input signal keeps its value during the time td.
      settings: CopyFcn=set_param(gcbh,'ShowName','off');
      mask Display: plot([0.4 0.7 0.7 0.8], [0.3 0.3 0.7 0.7])
  SignalTurnOnOffDelay : Subsystem  mask(GL_SignalDelayEither_1.0){}
      mask help: Signal delay. Delays a logical change the time td. The output signal will not change unless the input signal keeps its value during the time td.
      settings: CopyFcn=set_param(gcbh,'ShowName','off');
      mask Display:
      | plot([0.4 0.7 0.7 0.8], [0.3 0.3 0.7 0.7]+0.3)
      | plot([0.4 0.7 0.7 0.8], [0.7 0.7 0.3 0.3]-0.3)
  Switch : Switch  Criteria=u2 ~= 0  OutDataTypeStr=Inherit: Inherit via back propagation  RndMeth=Round
      mask init:
      | set_param(gcb, 'LinkStatus', 'none');
      | % 这句的使用场景：
      | % 当模型没有这句时，模型传递给没有模型库的人员会出现红色的错误框
      | % 没有模型库的使用者不能查看此模块
      settings: CopyFcn=set_param(gcb,'showname','off');
      mask Display:
      | plot([0.54 0.65],[0.92 0.92])
      | plot([0.6 0.6],[0.84 0.92])
      | 
      | plot([0.54 0.54],[0.05 0.14])
      | plot([0.54 0.65],[0.14 0.14])
      | plot([0.54 0.625],[0.08 0.08])
  xbackground1 : Subsystem
      mask Display: disp(' ')
  xbackground10 : UXFD_Lib/Standard/Relation&Logic/xbackground6  SystemSampleTime=-1  VariantActivationTime=update diagram  Latency=0  AutoFrameSizeCalculation=off
  xbackground2 : Subsystem
      mask Display: disp(' ')
  xbackground3 : Subsystem
      mask Display: disp(' ')
  xbackground4 : Subsystem
      mask Display: disp(' ')
  xbackground5 : Subsystem
      mask Display: disp(' ')
  xbackground6 : Subsystem
      mask Display: disp(' ')
  xbackground7 : Subsystem
      mask Display: disp(' ')
  xbackground8 : Subsystem
      mask Display: disp(' ')
  xbackground9 : Subsystem
      mask Display: disp(' ')

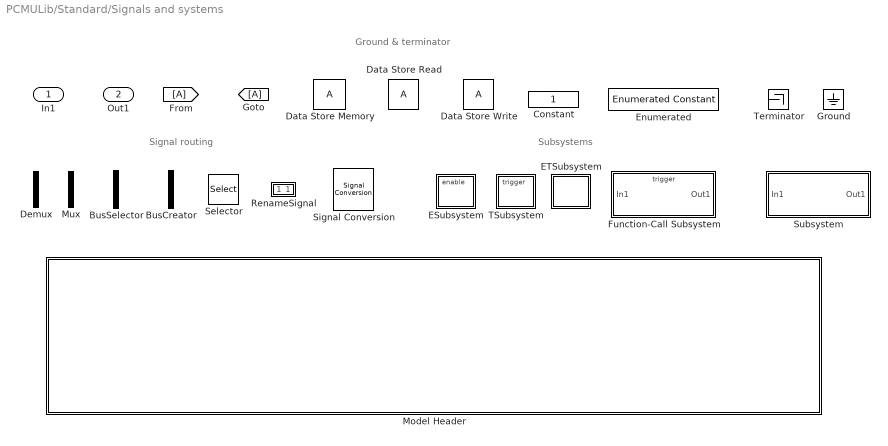
== system PCMULib/Standard/Signals and systems ==
  note: Subsystems
  note: Ground & terminator
  note: Signal routing
  In1 : Inport
  BusCreator : BusCreator  Inputs=2
      settings: CopyFcn=set_param(gcbh,'ShowName','off');
  BusSelector : BusSelector  OutputSignals=signal1,signal2
      settings: CopyFcn=set_param(gcbh,'ShowName','off');
  Constant : Constant  OutDataTypeStr=Inherit: Inherit via back propagation
      settings: CopyFcn=set_param(gcbh,'ShowName','off');
  Data Store Memory : DataStoreMemory  ReadBeforeWriteMsg=warning  WriteAfterWriteMsg=warning  WriteAfterReadMsg=warning  ShowAdditionalParam=off
      settings: CopyFcn=set_param(gcbh,'ShowName','off');
  Data Store Read : DataStoreRead  IndexOptions=Index vector (dialog)  Indices=1  OutputSizes=1
      settings: CopyFcn=set_param(gcbh,'ShowName','off');
  Data Store Write : DataStoreWrite  IndexOptions=Index vector (dialog)  Indices=1  OutputSizes=1
      settings: CopyFcn=set_param(gcbh,'ShowName','off');
  Demux : Demux  Outputs=3
      settings: CopyFcn=set_param(gcbh,'ShowName','off');  DisplayOption=none
  ESubsystem : Subsystem  TreatAsAtomicUnit=on
      mask init:
      | set_param(gcb, 'LinkStatus', 'none');
      mask Display: disp(' ');
  ETSubsystem : Subsystem  TreatAsAtomicUnit=on
      mask init:
      | set_param(gcb, 'LinkStatus', 'none');
      mask Display: disp(' ');
  Enumerated : simulink/Sources/Enumerated Constant  OutDataTypeStr=Enum: SlDemoSign  Value=SlDemoSign.Positive  SampleTime=inf
  From : From
      settings: CopyFcn=set_param(gcbh,'ShowName','off');
  Function-Call Subsystem : Subsystem  TreatAsAtomicUnit=on
      mask init:
      | set_param(gcb, 'LinkStatus', 'none');
  Goto : Goto
      settings: CopyFcn=set_param(gcbh,'ShowName','off');
  Ground : Ground
      settings: CopyFcn=set_param(gcbh,'ShowName','off');
  Model Header : Subsystem  mask(ModelHeader){prj='48V XXXXX', desc='Model Description', ver='V1.0.1', date='2017. 10. 12', rev='0', author=' '}
      mask prompts: prj "Project"; desc "Description"; ver "Version"
      mask init:
      | set_param(gcb, 'LinkStatus', 'none');
      settings: CopyFcn=set_param(gcbh,'ShowName','off');
      mask Display:
      | plot([0 0 1 1 0],[0.03 1 1 0.03 0.03])
      | plot([0 1],[0.4 0.4])
      | plot([0.5 0.5],[0.4 1])
      | plot([0.59 0.59],[0.4 1])
      | plot([0.5 1],[0.8 0.8])
      | plot([0.5 1],[0.6 0.6])
      | plot([0.75 0.75],[0.4 1])
      | plot([0.82 0.82],[0.6 1])
      | plot([0.75 0.75],[0.6 0.8])
      | plot([0.82 0.82],[0.4 0.8])
      | image(imread('geely.png','png'),[0.16 0.43 0.15 0.53])
      | text(0.01,0.34,['\fontsize{14}\fontname{Times}\bfPROPRIETARY AND CONFIDENTIAL:\rm\fontsize{11}\newline\it\fontsize{13}\fontname{Arial}'                 '    The Information Contained In This Model Is The Property Of Geely Automobile Research Institute. All Right Reserved.'                 ],'verticalAlignment','Top','horizontalAlignment','Left','texmode','on');
      | text(0.51,0.96,['\fontsize{14}\fontname{Times}\bfProject:       \rm\fontsize{11}\fontsize{12}' prj],'verticalAlignment','Top','horizontalAlignment','Left','texmode','on');
      | text(0.51,0.77,['\fontsize{14}\fontname{Times}\bfVersion:       \rm\fontsize{11}\fontsize{12}' ver],'verticalAlignment','Top','horizontalAlignment','Left','texmode','on');
      | text(0.51,0.56,['\fontsize{14}\fontname{Times}\bfDate:           \rm\fontsize{11}\fontsize{12}' date],'verticalAlignment','Top','horizontalAlignment','Left','texmode','on');
      | text(0.76,0.56,['\fontsize{14}\fontname{Times}\bfModel:    \rm\fontsize{11}\fontsize{12}' desc],'verticalAlignment','Top','horizontalAlignment','Left','texmode','on');
      | text(0.76,0.77,['\fontsize{14}\fontname{Times}\bfRev:        \rm\fontsize{11}\fontsize{12}' rev],'verticalAlignment','Top','horizontalAlignment','Left','texmode','on');
      | text(0.76,0.96,['\fontsize{14}\fontname{Times}\bfAuthor:    \rm\fontsize{11}\fontsize{12}' author],'verticalAlignment','Top','horizontalAlignment','Left','texmode','on');
  Mux : Mux  Inputs=3
      settings: CopyFcn=set_param(gcbh,'ShowName','off');
  RenameSignal : Subsystem  mask(GL_RenameSignal_1.0){}
      mask help: This block should be used to rename signals.
      mask init:
      | set_param(gcb, 'LinkStatus','none');
      settings: CopyFcn=set_param(gcbh,'ShowName','off');
      mask Display:
      | plot([0,1],[0.5,0.5]);
      | patch([0.2, 0.5, 0.2], [0.0,0.5, 1]);
      | patch([0.6, 0.9, 0.6], [0.0,0.5, 1]);
      | plot([0, 1, 1, 0, 0], [0, 0, 1, 1, 0])
  Selector : Selector  InputPortWidth=3  IndexOptions=Index vector (dialog)  Indices=[1 3]  OutputSizes=1
      settings: CopyFcn=set_param(gcbh,'ShowName','off');
  Signal Conversion : SignalConversion  ConversionOutput=Contiguous copy  OverrideOpt=off
      settings: CopyFcn=set_param(gcbh,'ShowName','off');
  Subsystem : Subsystem
  TSubsystem : Subsystem  TreatAsAtomicUnit=on
      mask init:
      | set_param(gcb, 'LinkStatus', 'none');
      mask Display: disp(' ');
  Terminator : Terminator
      settings: CopyFcn=set_param(gcbh,'ShowName','off');
  Out1 : Outport  Port=2
